simulink model "simulation"  (Simulink 8.6)
settings: Solver=VariableStepAuto  StartTime=0.0  StopTime=100  RelTol=1e-3
values from neighbouring files (symbols this model uses):
  bDevice = block.DialogPrm(1).Data    [Controller.m]    (also in Controller1.m; LessConservative.m; MoreConservative.m; Parameters.m = 0.1)
  mDevice = 0.1    [Parameters.m]
  p0 = block.DialogPrm(4).Data    [Controller.m]    (also in Controller1.m; Initiation.m = 0.12; Parameters.m = 1; VirtualEnvironment.m = block.DialogPrm(8).Data)
  v0 = block.DialogPrm(6).Data    [HapticDevice.m]    (also in HumanOperator.m; Initiation.m = 0; Parameters.m = 0; VirtualEnvironment4.m = block.DialogPrm(8).Data)
settings Model: Creator=TOSHIBA  LastModifiedBy=TOSHIBA
settings DataIOCC: SaveFormat=Dataset  SignalLoggingSaveFormat=Dataset
settings OptimizationCC: ExpressionDepthLimit=128
settings DebuggingCC: UnderspecifiedInitializationDetection=Simplified  MergeDetectMultiDrivingBlocksExec=error  SolverPrmCheckMsg=none  FcnCallInpInsideContextMsg=EnableAllAsError  StateNameClashWarn=none
settings HardwareCC: ProdBitPerPointer=64  ProdLargestAtomicFloat=Float  ProdIntDivRoundTo=Zero  ProdEndianess=LittleEndian  ProdWordSize=64  ProdHWDeviceType=Intel->x86-64 (Windows64)
settings GRTTargetCC: GeneratePreprocessorConditionals=Use local settings  CombineOutputUpdateFcns=on  GRTInterface=off
settings ConfigComp: CovModelRefEnable=off

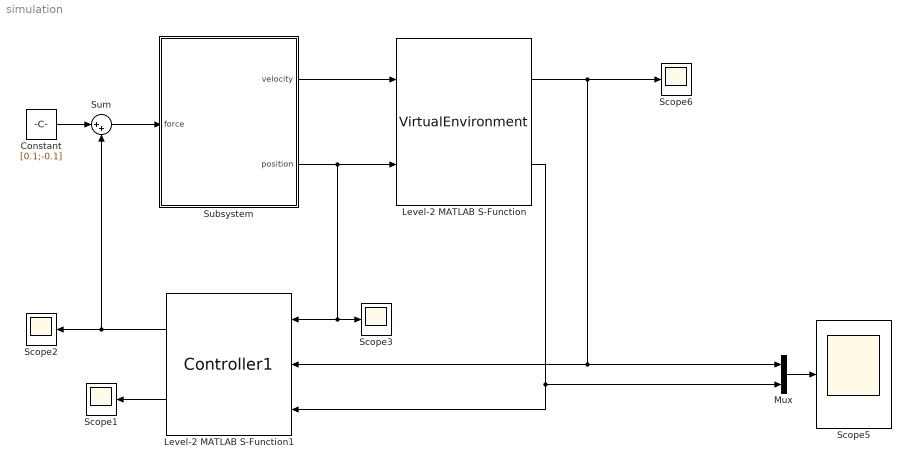
== system simulation ==
  Constant : Constant  Value=[0.1;-0.1]
  Level-2 MATLAB S-Function : M-S-Function  FunctionName=VirtualEnvironment  Parameters=kWall, bWall, nWall, pWall, mu, dof, tsampling
  Level-2 MATLAB S-Function1 : M-S-Function  FunctionName=Controller1  Parameters=bDevice, dof, tsampling, p0, pWall, nWall
  Mux : Mux  Inputs=2
  Scope{1..3,5..6} (5 alike) : Scope
  Subsystem : Subsystem
  Sum : Sum  Inputs=|++
  wires:
  Sum/1 -> Subsystem/1(force)
  Subsystem/1(velocity) -> Level-2 MATLAB S-Function/1
  Subsystem/2(position) -> Scope3/1, Level-2 MATLAB S-Function1/1, Level-2 MATLAB S-Function/2
  Constant/1 -> Sum/1
  Level-2 MATLAB S-Function1/1 -> Sum/2, Scope2/1
  Level-2 MATLAB S-Function1/2 -> Scope1/1
  Mux/1 -> Scope5/1
  Level-2 MATLAB S-Function/1 -> Scope6/1, Mux/1, Level-2 MATLAB S-Function1/2
  Level-2 MATLAB S-Function/2 -> Mux/2, Level-2 MATLAB S-Function1/3

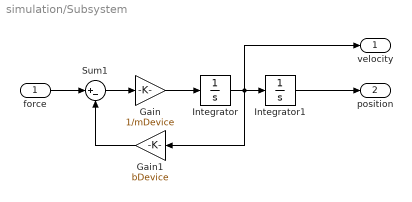
== system simulation/Subsystem ==
  force : Inport
  Gain : Gain  Gain=1/mDevice
  Gain1 : Gain  Gain=bDevice
  Integrator : Integrator  InitialCondition=v0
  Integrator1 : Integrator  InitialCondition=p0
  Sum1 : Sum  Inputs=|+-
  velocity : Outport
  position : Outport  Port=2
  wires:
  Gain1/1 -> Sum1/2
  force/1 -> Sum1/1
  Sum1/1 -> Gain/1
  Integrator/1 -> velocity/1, Gain1/1, Integrator1/1
  Gain/1 -> Integrator/1
  Integrator1/1 -> position/1
